simulink model "practica5"  (R2019b)
settings: Solver=FixedStepAuto  StartTime=0.0  StopTime=10.0  RelTol=1e-3  EnableMultiTasking=on
undefined symbols (not defined in the file): t_sim
libraries: legoev3lib x4, simulink x1
settings Model: ExtModeTrigDuration=2  Creator=alumnopr09  LastModifiedBy=alumnopr09
settings SolverCC: PositivePriorityOrder=on
settings OptimizationCC: EnhancedBackFolding=on  PassReuseOutputArgsAs=Individual arguments  ZeroExternalMemoryAtStartup=off  ZeroInternalMemoryAtStartup=off  MaxStackSize=64  OptimizeBlockOrder=speed  DifferentSizesBufferReuse=on  OptimizationCustomize=off  EfficientTunableParamExpr=on
settings DebuggingCC: ParameterTunabilityLossMsg=error
settings HardwareCC: ProdBitPerPointer=32  ProdBitPerSizeT=32  ProdBitPerPtrDiffT=32  ProdLargestAtomicInteger=Long  ProdWordSize=32  ProdHWDeviceType=ARM Compatible->ARM 9
settings SFSimCC: MATLABDynamicMemAlloc=off
settings RTWCC: SystemTargetFile=ert.tlc  HardwareBoard=LEGO MINDSTORMS EV3  TLCOptions="-aInlineSetEventsForThisBaseRateFcn=TLC_FALSE -aSuppressMultiTaskScheduler=TLC_FALSE  -aRateBasedStepFcn=0"  TemplateMakefile=ert_default_tmf  GenerateReport=on  Toolchain=Sourcery G++ Lite v2009q3  IncludeHyperlinkInReport=on  LaunchReport=on  GenerateTraceInfo=on  GenerateTraceReport=on  GenerateTraceReportSl=on  GenerateTraceReportSf=on  GenerateTraceReportEml=on
settings CodeAppCC: ForceParamTrailComments=on  IgnoreCustomStorageClasses=off  OperatorAnnotations=on  SimulinkDataObjDesc=on  SFDataObjDesc=on  InsertBlockDesc=on
settings ERTTargetCC: SupportContinuousTime=on  SupportVariableSizeSignals=on

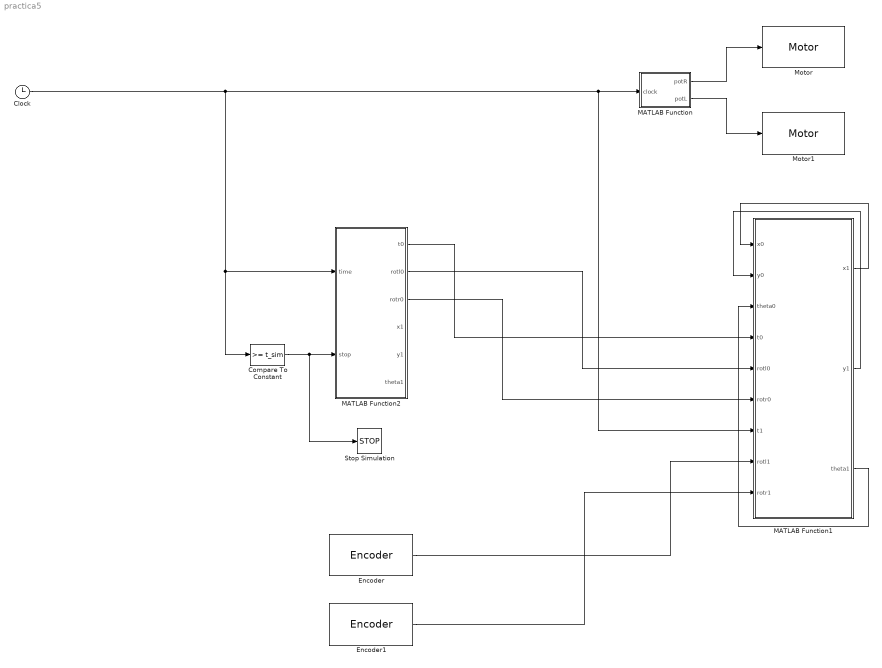
== system practica5 ==
  Clock : Clock
  Compare To Constant : simulink/Logic and Bit Operations/Compare To Constant  relop=>=  const=t_sim  OutDataTypeStr=boolean
  Encoder : legoev3lib/Encoder  portNumber=A  opMode=Reset at each sample time  sampleTime=0.1
      settings: SourceProductName=Simulink Support Package for LEGO MINDSTORMS EV3 Hardware  SourceProductBaseCode=LEGOEV3
  Encoder1 : legoev3lib/Encoder  portNumber=D  opMode=Reset at each sample time  sampleTime=0.1
      settings: SourceProductName=Simulink Support Package for LEGO MINDSTORMS EV3 Hardware  SourceProductBaseCode=LEGOEV3
  MATLAB Function : MATLAB Function  TreatAsAtomicUnit=on
  MATLAB Function1 : MATLAB Function  TreatAsAtomicUnit=on
  MATLAB Function2 : MATLAB Function  TreatAsAtomicUnit=on
  Motor : legoev3lib/Motor  sportNumber=D  sstopAction=Brake
  Motor1 : legoev3lib/Motor  sportNumber=A  sstopAction=Brake
  Stop Simulation : Stop
  wires:
  MATLAB Function/1(potR) -> Motor/1
  MATLAB Function/2(potL) -> Motor1/1
  Encoder/1 -> MATLAB Function1/8(rotl1)
  Encoder1/1 -> MATLAB Function1/9(rotr1)
  Clock/1 -> Compare To Constant/1, MATLAB Function2/1(time), MATLAB Function1/7(t1), MATLAB Function/1(clock)
  Compare To Constant/1 -> Stop Simulation/1, MATLAB Function2/2(stop)
  MATLAB Function2/1(t0) -> MATLAB Function1/4(t0)
  MATLAB Function2/2(rotl0) -> MATLAB Function1/5(rotl0)
  MATLAB Function2/3(rotr0) -> MATLAB Function1/6(rotr0)
  MATLAB Function1/1(x1) -> MATLAB Function1/1(x0)
  MATLAB Function1/2(y1) -> MATLAB Function1/2(y0)
  MATLAB Function1/3(theta1) -> MATLAB Function1/3(theta0)

== matlab function practica5/MATLAB Function1 ==
  data: x0 input; x1 output; y0 input; theta0 input; t0 input; rotl0 input; rotr0 input; t1 input; rotl1 input; rotr1 input; y1 output; theta1 output
function [x1,y1,theta1]=odometry(x0,y0,theta0,t0,rotl0,rotr0,t1,rotl1,rotr1)
    D = 11.7;
    R = 2.7;
    deltaThetaL = rotl1 - rotl0;
    deltaThetaR = rotr1 - rotr0;
    deltaTiempo = t1 - t0;
    
    if deltaTiempo == 0
        x1 = x0;
        y1 = y0;
        theta1 = theta0;
    else
    	x1 = (deltaThetaL * R) + (deltaThetaR * R) / 2 * cos(theta0);
    	y1 = (deltaThetaL * R) + (deltaThetaR * R) / 2 * sin(theta0);
    	theta1 = (deltaThetaR * R) - (deltaThetaL * R) / D;
    end
       
end

== matlab function practica5/MATLAB Function ==
  data: potR output; potL output; clock input
function [potR, potL] = fcn(clock)

    %Constantes generales
    P = 50; % potencia de las ruedas
    t_recta = 1.5 % tiempo en hacer una linea recta
    t_giro = 1 % tiempo en girar
  
    persistent ultimotiempo
    if (isempty(ultimotiempo))
        ultimotiempo = 0;
    end
    
    persistent estado
    if (isempty(estado))
        estado = false; % 0 --> Recto; 1 --> Giro
    end
    
    persistent total_time; % tiempo en segundos
    if (isempty(total_time))
        total_time = 0;
    end
    
    %Variables utiles
    Radio = 2.7 % cm
    Dist_Ruedas = 11.7 % cm

    % -------------------------
    % DESARROLLO DE LA PRACTICA
    % -------------------------

    deltat = clock-ultimotiempo;
    if (not(estado))
        % Mover en linea recta:
        potR = P;
        potL = P;
        total_time = total_time + deltat ;
        if (total_time > t_recta)
            total_time = 0;
            estado = true;
        end
    else
        % Girar a la derecha:
        potR = 0;
        potL = P;
        total_time = total_time + deltat ;
        if (total_time > t_giro)
            total_time = 0;
            estado = false;
        end
    end
ultimotiempo = clock;

== matlab function practica5/MATLAB Function2 ==
  data: time input; stop input; t0 output; rotl0 output; rotr0 output; x1 output; y1 output; theta1 output
function [t0,rotl0,rotr0,x1,y1,theta1] = logger (time,stop)
persistent myFile;

if (isempty(myFile))
    myFile= fopen('C:\Users\alumnopr09\Downloads\','r');
end

if(myFile>=0)
    if(stop>0)
        fclose(myFile);
    else
        %Imprimimos los datos dentro del archivo
        a = fscanf(myFile,'%f\t%i\n',time,int32(light));
        t0=a(0,1);
        rotl0=a(0,2);
        rotr0=a(0,3);
        x1=a(0,4);
        y1=a(0,5);
        theta1=a(0,6);
    end
end
